simulink model "cvoo_g19_at_sens_est_bombom"  (R2020a)
settings: Solver=VariableStepAuto  StartTime=0.0  StopTime=100  RelTol=1e-3
values from neighbouring files (symbols this model uses):
  b_h_pt = [ ... (first row only)    [main.m]
  c_h_pt = eye(size(a_h_pt))    [main.m]
  conv_max = 5    [main.m]
  conv_min = 0    [main.m]
  conv_rms = 1.5*conv_res    (= 0.000915639116103)    [main.m]
  d_h_pt = zeros(size(b_h_pt))    [main.m]
  deg = pi/180    (= 0.0174532925199)    [main.m]    (also in main_gaspar.m)
  f_amost = 100    [main.m]
  fat_conv_ra = 1/3    (= 0.333333333333)    [main.m]
  G_ra = 10e-3/ft    (= 0.0328083989501)    [main.m]
  G_sensq = (V_max_sensq-V_min_sensq)/(q_max_sensq-q_min_sensq)    (= 0.006)    [main.m]
  Gp_din = (v_pdin_max-v_pdin_min)/(pdin_max-pdin_min)    (= 0.00125)    [main.m]
  h_pt_ref = -1    [main.m]    (also in main_gaspar.m)
  h_ra_max = 1500*ft    (= 457.2)    [main.m]
  h_ra_min = 0    [main.m]
  h_ref = fscanf(fileID,'    [ground_model.m]
  K_lqr = lqr(a_h_pt_int, b_h_pt_int, Q, R)    [main.m]    (also in main_gaspar.m = lqr(a_h_int, b_h_sf_int, Q, R))
  offset_alt = 200    [main.m]
  offset_pdin = 2.5    [main.m]
  Offset_ra = 0    [main.m]
  Offset_sensq = 2.5    [main.m]
  p_din_tau = 0.01    [main.m]
  pdin_max = 2e3    (= 2000)    [main.m]
  pdin_min = -2e3    (= -2000)    [main.m]
  q_max_sensq = 300    [main.m]
  q_min_sensq = -300    [main.m]
  ra_rms = 0.015    [main.m]
  rad = 180/pi    (= 57.2957795131)    [main.m]    (also in main_gaspar.m)
  rho0 = 1.225    [main.m]
  rms_sensq = 4.4    [main.m]
  tau = 0.1    [main.m]
  u_ref = 2    [main.m]    (also in main_gaspar.m = -5)
  vel_max_at = 60    [main.m]
  x0 = [0 0 0 0]    [main.m]    (also in main_gaspar.m)
  x0_e = [0 0 0 0 0]    [main.m]
undefined symbols (not defined in the file or in its folder): a_h_pt, ae, be, ce, cond_ini, de, max_deflec
libraries: simulink x5
settings Model: Creator=josem  LastModifiedBy=thomasmchilds

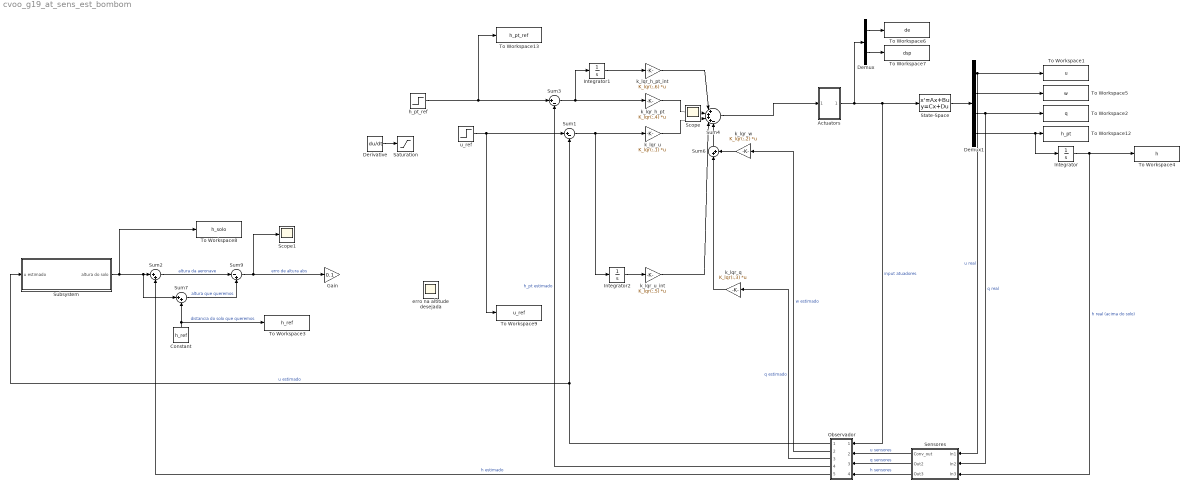
== system cvoo_g19_at_sens_est_bombom ==
  Actuators : Subsystem
  Constant : Constant  Value=h_ref
  Demux : Demux  Outputs=2
  Demux1 : Demux
  Derivative : Derivative
  Gain : Gain  Gain=0.1
  Integrator : Integrator  InitialCondition=cond_ini.h0
  Integrator1 : Integrator
  Integrator2 : Integrator
  Observador : Subsystem
  Saturation : Saturate  UpperLimit=10  LowerLimit=-10
  Scope1 : Scope
  Sensores : Subsystem
  State-Space : StateSpace  A=a_h_pt  B=b_h_pt  C=c_h_pt  D=d_h_pt  InitialCondition=x0
  Subsystem : Subsystem
  Sum1 : Sum  Inputs=|+-
  Sum2 : Sum  Inputs=|++
  Sum3 : Sum  Inputs=|+-
  Sum4 : Sum  Inputs=|++++-
  Sum6 : Sum  Inputs=|++
  Sum7 : Sum  Inputs=|++
  Sum9 : Sum  Inputs=|-+
  To Workspace1 : ToWorkspace  VariableName=u  SampleTime=-1
  To Workspace12 : ToWorkspace  VariableName=h_pt  SampleTime=-1
  To Workspace13 : ToWorkspace  VariableName=h_pt_ref  SampleTime=-1
  To Workspace2 : ToWorkspace  VariableName=q  SampleTime=-1
  To Workspace3 : ToWorkspace  VariableName=h_ref  SampleTime=-1
  To Workspace4 : ToWorkspace  VariableName=h  SampleTime=-1
  To Workspace5 : ToWorkspace  VariableName=w  SampleTime=-1
  To Workspace6 : ToWorkspace  VariableName=de  SaveFormat=Structure With Time  SampleTime=-1
  To Workspace7 : ToWorkspace  VariableName=dsp  SaveFormat=Structure With Time  SampleTime=-1
  To Workspace8 : ToWorkspace  VariableName=h_solo  SampleTime=-1
  To Workspace9 : ToWorkspace  VariableName=u_ref  SampleTime=-1
  erro na altitude desejada : Scope
  h_pt_ref : Step  Time=10  After=h_pt_ref  SampleTime=0  VectorParams1D=off
  k_lqr_h_pt : Gain  Gain=K_lqr(:,4)  Multiplication=Matrix(K*u)
  k_lqr_h_pt_int : Gain  Gain=K_lqr(:,6)  Multiplication=Matrix(K*u)
  k_lqr_q : Gain  Gain=K_lqr(:,3)  Multiplication=Matrix(K*u)
  k_lqr_u : Gain  Gain=K_lqr(:,1)  Multiplication=Matrix(K*u)
  k_lqr_u_int : Gain  Gain=K_lqr(:,5)  Multiplication=Matrix(K*u)
  k_lqr_w : Gain  Gain=K_lqr(:,2)  Multiplication=Matrix(K*u)
  u_ref : Step  Time=50  After=u_ref  SampleTime=0  VectorParams1D=off
  Scope : Scope
  wires:
  State-Space/1 -> Demux1/1
  Demux1/2 -> To Workspace5/1
  k_lqr_h_pt/1 -> Sum4/2
  k_lqr_w/1 -> Sum6/2
  k_lqr_q/1 -> Sum6/1
  Sum6/1 -> Sum4/5
  Demux/1 -> To Workspace6/1
  Demux/2 -> To Workspace7/1
  Demux1/4 -> Integrator/1, To Workspace12/1
  Demux1/1 -> To Workspace1/1, Sensores/1(In1)  "u real"
  k_lqr_u/1 -> Sum4/3
  Sum3/1 -> Integrator1/1, k_lqr_h_pt/1
  Integrator1/1 -> k_lqr_h_pt_int/1
  k_lqr_h_pt_int/1 -> Sum4/1
  k_lqr_u_int/1 -> Sum4/4
  Sum1/1 -> Integrator2/1, k_lqr_u/1
  Integrator2/1 -> k_lqr_u_int/1
  Sum4/1 -> Actuators/1(In1)
  Actuators/1(Out1) -> State-Space/1, Observador/1(In1), Demux/1  "input atuadores"
  Demux1/3 -> To Workspace2/1, Sensores/2(In2)  "q real"
  u_ref/1 -> To Workspace9/1, Sum1/1
  Integrator/1 -> Sensores/3(In3), To Workspace4/1  "h real (acima do solo)"
  Observador/1(Out4) -> Subsystem/1(u estimado), Sum1/2  "u estimado"
  Observador/4(Out1) -> Sum3/2  "h_pt estimado"
  Observador/2(Out2) -> k_lqr_w/1  "w estimado"
  Observador/3(Out3) -> k_lqr_q/1  "q estimado"
  Sensores/1(Conv_out) -> Observador/2(In2)  "u sensores"
  Sensores/2(Out2) -> Observador/3(In3)  "q sensores"
  Sensores/3(Out3) -> Observador/4(In4)  "h sensores"
  Observador/5(Out5) -> Sum2/2  "h estimado"
  Derivative/1 -> Saturation/1
  Sum9/1 -> Scope1/1, Gain/1  "erro de altura abs"
  Sum2/1 -> Sum9/1  "altura da aeronave"
  Subsystem/1(altura do solo) -> To Workspace8/1, Sum7/1, Sum2/1
  Constant/1 -> Sum7/2, To Workspace3/1  "distancia do solo que queremos"
  Sum7/1 -> Sum9/2  "altura que queremos"
  h_pt_ref/1 -> To Workspace13/1, Sum3/1

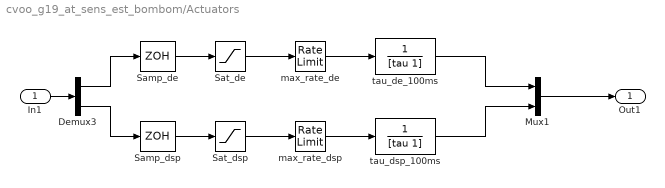
== system cvoo_g19_at_sens_est_bombom/Actuators ==
  In1 : Inport
  " max_rate_de" : RateLimiter  RisingSlewLimit=vel_max_at*deg  FallingSlewLimit=-vel_max_at*deg  SampleTimeMode=inherited
  " max_rate_dsp" : RateLimiter  RisingSlewLimit=vel_max_at*deg  FallingSlewLimit=-vel_max_at*deg  SampleTimeMode=inherited
  Demux3 : Demux  Outputs=2
  Mux1 : Mux  Inputs=2
  Samp_de : ZeroOrderHold  SampleTime=1/f_amost
  Samp_dsp : ZeroOrderHold  SampleTime=1/f_amost
  Sat_de : Saturate  UpperLimit=max_deflec.demax  LowerLimit=max_deflec.demin
  Sat_dsp : Saturate  UpperLimit=max_deflec.spmax  LowerLimit=0
  tau_de_100ms : TransferFcn  Denominator=[tau 1]
  tau_dsp_100ms : TransferFcn  Denominator=[tau 1]
  Out1 : Outport
  wires:
  Mux1/1 -> Out1/1
  In1/1 -> Demux3/1
  Sat_dsp/1 -> " max_rate_dsp"/1
  Sat_de/1 -> " max_rate_de"/1
  Demux3/1 -> Samp_de/1
  Demux3/2 -> Samp_dsp/1
  Samp_dsp/1 -> Sat_dsp/1
  Samp_de/1 -> Sat_de/1
  " max_rate_de"/1 -> tau_de_100ms/1
  " max_rate_dsp"/1 -> tau_dsp_100ms/1
  tau_dsp_100ms/1 -> Mux1/2
  tau_de_100ms/1 -> Mux1/1

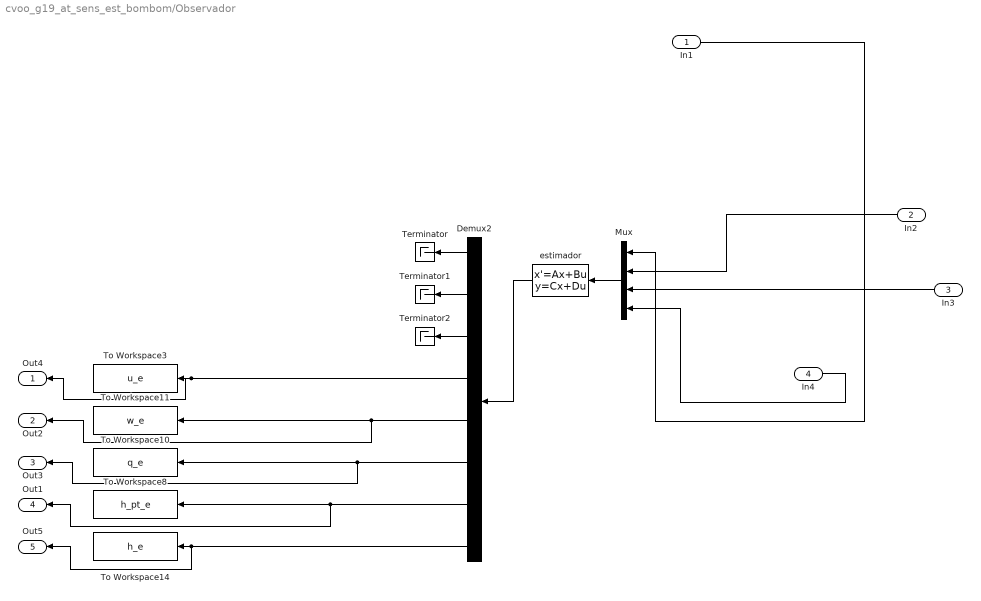
== system cvoo_g19_at_sens_est_bombom/Observador ==
  In1 : Inport
  In2 : Inport  Port=2
  In3 : Inport  Port=3
  In4 : Inport  Port=4
  Demux2 : Demux  Outputs=8
  Mux : Mux
  Terminator : Terminator
  Terminator1 : Terminator
  Terminator2 : Terminator
  To Workspace10 : ToWorkspace  VariableName=q_e  SampleTime=-1
  To Workspace11 : ToWorkspace  VariableName=w_e  SampleTime=-1
  To Workspace14 : ToWorkspace  VariableName=h_e  SampleTime=-1
  To Workspace3 : ToWorkspace  VariableName=u_e  SampleTime=-1
  To Workspace8 : ToWorkspace  VariableName=h_pt_e  SampleTime=-1
  estimador : StateSpace  A=ae  B=be  C=ce  D=de  InitialCondition=x0_e
  Out4 : Outport
  Out2 : Outport  Port=2
  Out3 : Outport  Port=3
  Out1 : Outport  Port=4
  Out5 : Outport  Port=5
  wires:
  Demux2/2 -> Terminator1/1
  estimador/1 -> Demux2/1
  Demux2/5 -> Out2/1, To Workspace11/1
  Demux2/7 -> Out1/1, To Workspace8/1
  Demux2/8 -> Out5/1, To Workspace14/1
  Demux2/1 -> Terminator/1
  Demux2/4 -> Out4/1, To Workspace3/1
  Demux2/3 -> Terminator2/1
  Mux/1 -> estimador/1
  Demux2/6 -> Out3/1, To Workspace10/1
  In1/1 -> Mux/1
  In3/1 -> Mux/3
  In2/1 -> Mux/2
  In4/1 -> Mux/4

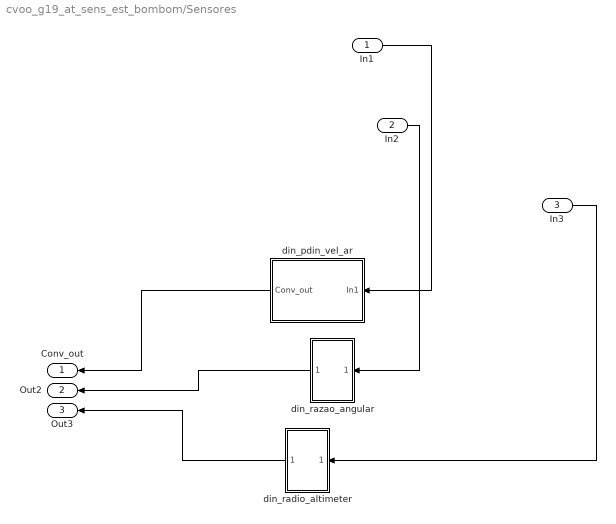
== system cvoo_g19_at_sens_est_bombom/Sensores ==
  In1 : Inport
  In2 : Inport  Port=2
  In3 : Inport  Port=3
  din_pdin_vel_ar : Subsystem
  din_radio_altimeter : Subsystem
  din_razao_angular : Subsystem
  Conv_out : Outport
  Out2 : Outport  Port=2
  Out3 : Outport  Port=3
  wires:
  din_razao_angular/1(Out1) -> Out2/1
  In1/1 -> din_pdin_vel_ar/1(In1)
  din_pdin_vel_ar/1(Conv_out) -> Conv_out/1
  In2/1 -> din_razao_angular/1(In1)
  In3/1 -> din_radio_altimeter/1(In1)
  din_radio_altimeter/1(Out1) -> Out3/1

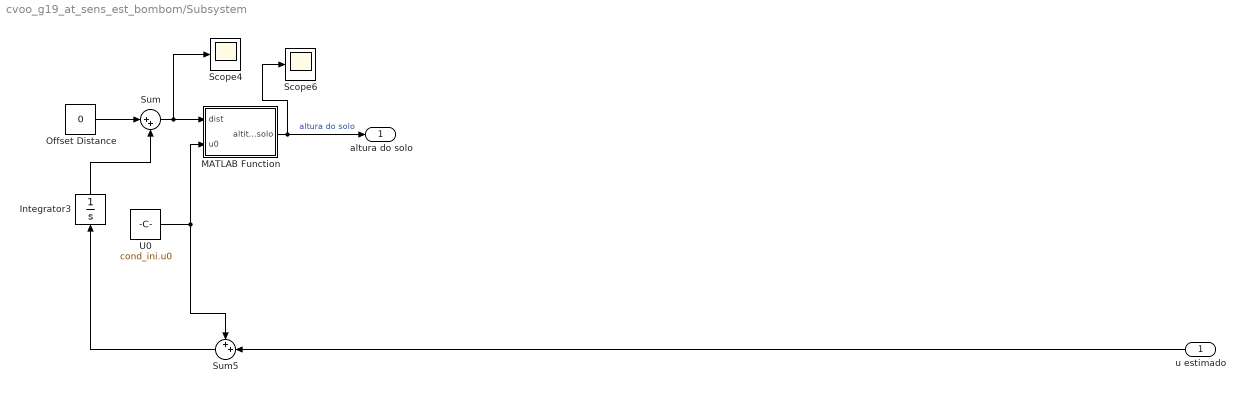
== system cvoo_g19_at_sens_est_bombom/Subsystem ==
  u estimado : Inport
  Integrator3 : Integrator
  MATLAB Function : MATLAB Function  TreatAsAtomicUnit=on
  Offset Distance : Constant  Value=0
  Scope4 : Scope
  Scope6 : Scope
  Sum : Sum  Inputs=|++
  Sum5 : Sum  Inputs=++|
  U0 : Constant  Value=cond_ini.u0
  altura do solo : Outport
  wires:
  Integrator3/1 -> Sum/2
  MATLAB Function/1(altitude_solo) -> altura do solo/1, Scope6/1  "altura do solo"
  Sum5/1 -> Integrator3/1
  U0/1 -> MATLAB Function/2(u0), Sum5/1
  Sum/1 -> Scope4/1, MATLAB Function/1(dist)
  u estimado/1 -> Sum5/2
  Offset Distance/1 -> Sum/1

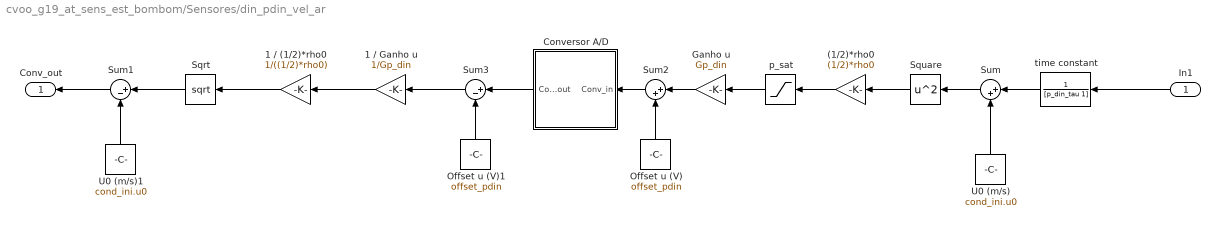
== system cvoo_g19_at_sens_est_bombom/Sensores/din_pdin_vel_ar ==
  In1 : Inport
  " time constant" : TransferFcn  Denominator=[p_din_tau 1]
  (1/2)*rho0 : Gain  Gain=(1/2)*rho0
  1 / (1/2)*rho0 : Gain  Gain=1/((1/2)*rho0)
  1 / Ganho u : Gain  Gain=1/Gp_din
  Conversor A/D : Subsystem
  Ganho u : Gain  Gain=Gp_din
  Offset u (V) : Constant  Value=offset_pdin
  Offset u (V)1 : Constant  Value=offset_pdin
  Sqrt : Sqrt  SaturateOnIntegerOverflow=on
  Square : Math  Operator=square  SignedPower=on  SaturateOnIntegerOverflow=on
  Sum : Sum  Inputs=|++
  Sum1 : Sum  Inputs=|+-
  Sum2 : Sum  Inputs=|++
  Sum3 : Sum  Inputs=|+-
  U0 (m/s) : Constant  Value=cond_ini.u0
  U0 (m/s)1 : Constant  Value=cond_ini.u0
  p_sat : Saturate  UpperLimit=pdin_max  LowerLimit=pdin_min
  Conv_out : Outport
  wires:
  In1/1 -> " time constant"/1
  Sum/1 -> Square/1
  Ganho u/1 -> Sum2/1
  Offset u (V)/1 -> Sum2/2
  " time constant"/1 -> Sum/1
  (1/2)*rho0/1 -> p_sat/1
  U0 (m/s)/1 -> Sum/2
  p_sat/1 -> Ganho u/1
  Square/1 -> (1/2)*rho0/1
  Sum2/1 -> Conversor A/D/1(Conv_in)
  Offset u (V)1/1 -> Sum3/2
  U0 (m/s)1/1 -> Sum1/2
  Sqrt/1 -> Sum1/1
  1 / (1/2)*rho0/1 -> Sqrt/1
  1 / Ganho u/1 -> 1 / (1/2)*rho0/1
  Sum3/1 -> 1 / Ganho u/1
  Conversor A/D/1(Conv_out) -> Sum3/1
  Sum1/1 -> Conv_out/1

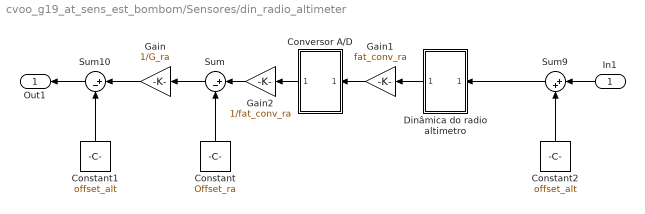
== system cvoo_g19_at_sens_est_bombom/Sensores/din_radio_altimeter ==
  In1 : Inport
  Constant : Constant  Value=Offset_ra
  Constant1 : Constant  Value=offset_alt
  Constant2 : Constant  Value=offset_alt
  Conversor A/D : Subsystem
  Dinâmica do radio altimetro : Subsystem
  Gain : Gain  Gain=1/G_ra
  Gain1 : Gain  Gain=fat_conv_ra
  Gain2 : Gain  Gain=1/fat_conv_ra
  Sum : Sum  Inputs=|+-
  Sum10 : Sum  Inputs=|+-
  Sum9 : Sum  Inputs=|++
  Out1 : Outport
  wires:
  Sum/1 -> Gain/1
  Constant/1 -> Sum/2
  Dinâmica do radio altimetro/1(Out1) -> Gain1/1
  Gain1/1 -> Conversor A/D/1(In1)
  Gain2/1 -> Sum/1
  Conversor A/D/1(Out1) -> Gain2/1
  Constant1/1 -> Sum10/2
  Gain/1 -> Sum10/1
  Sum10/1 -> Out1/1
  Constant2/1 -> Sum9/2
  In1/1 -> Sum9/1
  Sum9/1 -> Dinâmica do radio altimetro/1(In1)

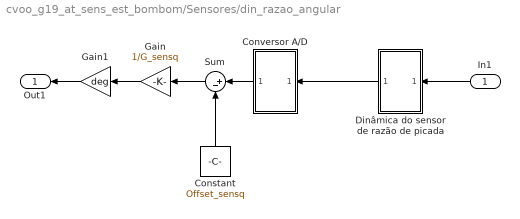
== system cvoo_g19_at_sens_est_bombom/Sensores/din_razao_angular ==
  In1 : Inport
  Constant : Constant  Value=Offset_sensq
  Conversor A/D : Subsystem
  Dinâmica do sensor de razão de picada : Subsystem
  Gain : Gain  Gain=1/G_sensq
  Gain1 : Gain  Gain=deg
  Sum : Sum  Inputs=|+-
  Out1 : Outport
  wires:
  In1/1 -> Dinâmica do sensor de razão de picada/1(In1)
  Dinâmica do sensor de razão de picada/1(Out1) -> Conversor A/D/1(In1)
  Conversor A/D/1(Out1) -> Sum/1
  Sum/1 -> Gain/1
  Constant/1 -> Sum/2
  Gain/1 -> Gain1/1
  Gain1/1 -> Out1/1

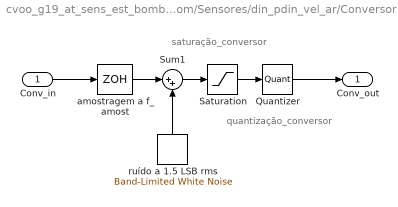
== system cvoo_g19_at_sens_est_bombom/Sensores/din_pdin_vel_ar/Conversor A//D ==
  note: saturação_conversor
  note: quantização_conversor
  Conv_in : Inport
  Quantizer : Quantizer  QuantizationInterval=fat_quant
  Saturation : Saturate  UpperLimit=conv_max  LowerLimit=conv_min
  Sum1 : Sum  Inputs=|++
  amostragem a f_amost : ZeroOrderHold  SampleTime=1/f_amost
  ruído a 1.5 LSB rms : simulink/Sources/Band-Limited White Noise  Cov=[conv_rms^2/f_amost]  Ts=1/f_amost  seed=[23341]
  Conv_out : Outport
  wires:
  Conv_in/1 -> amostragem a f_amost/1
  amostragem a f_amost/1 -> Sum1/1
  ruído a 1.5 LSB rms/1 -> Sum1/2
  Saturation/1 -> Quantizer/1
  Sum1/1 -> Saturation/1
  Quantizer/1 -> Conv_out/1

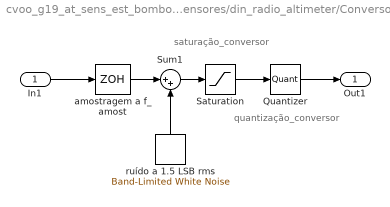
== system cvoo_g19_at_sens_est_bombom/Sensores/din_radio_altimeter/Conversor A//D ==
  note: saturação_conversor
  note: quantização_conversor
  In1 : Inport
  Quantizer : Quantizer  QuantizationInterval=fat_quant
  Saturation : Saturate  UpperLimit=conv_max  LowerLimit=conv_min
  Sum1 : Sum  Inputs=|++
  amostragem a f_amost : ZeroOrderHold  SampleTime=1/f_amost
  ruído a 1.5 LSB rms : simulink/Sources/Band-Limited White Noise  Cov=[conv_rms^2/f_amost]  Ts=1/f_amost  seed=[23341]
  Out1 : Outport
  wires:
  In1/1 -> amostragem a f_amost/1
  amostragem a f_amost/1 -> Sum1/1
  ruído a 1.5 LSB rms/1 -> Sum1/2
  Saturation/1 -> Quantizer/1
  Sum1/1 -> Saturation/1
  Quantizer/1 -> Out1/1

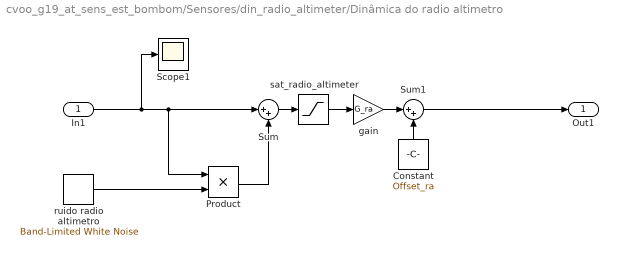
== system cvoo_g19_at_sens_est_bombom/Sensores/din_radio_altimeter/Dinâmica do radio altimetro ==
  In1 : Inport
  Constant : Constant  Value=Offset_ra
  Product : Product
  Scope1 : Scope
  Sum : Sum  Inputs=|++
  Sum1 : Sum  Inputs=|++
  gain : Gain  Gain=G_ra
  ruido radio altimetro : simulink/Sources/Band-Limited White Noise  Cov=[ra_rms^2/f_amost]  Ts=1/f_amost  seed=[23341]
  sat_radio_altimeter : Saturate  UpperLimit=h_ra_max  LowerLimit=h_ra_min
  Out1 : Outport
  wires:
  Sum1/1 -> Out1/1
  Sum/1 -> sat_radio_altimeter/1
  Constant/1 -> Sum1/2
  gain/1 -> Sum1/1
  sat_radio_altimeter/1 -> gain/1
  In1/1 -> Scope1/1, Sum/1, Product/1
  ruido radio altimetro/1 -> Product/2
  Product/1 -> Sum/2

== system cvoo_g19_at_sens_est_bombom/Sensores/din_razao_angular/Conversor A//D ==
  note: saturação_conversor
  note: quantização_conversor
  In1 : Inport
  Quantizer : Quantizer  QuantizationInterval=fat_quant
  Saturation : Saturate  UpperLimit=conv_max  LowerLimit=conv_min
  Sum1 : Sum  Inputs=|++
  amostragem a f_amost : ZeroOrderHold  SampleTime=1/f_amost
  ruído a 1.5 LSB rms : simulink/Sources/Band-Limited White Noise  Cov=[conv_rms^2/f_amost]  Ts=1/f_amost  seed=[23341]
  Out1 : Outport
  wires:
  In1/1 -> amostragem a f_amost/1
  amostragem a f_amost/1 -> Sum1/1
  ruído a 1.5 LSB rms/1 -> Sum1/2
  Saturation/1 -> Quantizer/1
  Sum1/1 -> Saturation/1
  Quantizer/1 -> Out1/1

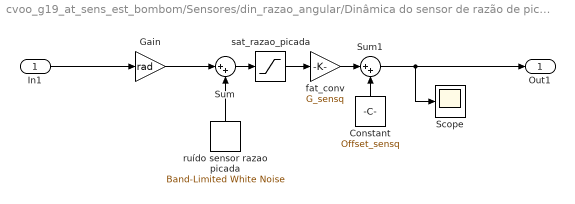
== system cvoo_g19_at_sens_est_bombom/Sensores/din_razao_angular/Dinâmica do sensor de razão de picada ==
  In1 : Inport
  Constant : Constant  Value=Offset_sensq
  Gain : Gain  Gain=rad
  Scope : Scope
  Sum : Sum  Inputs=|++
  Sum1 : Sum  Inputs=|++
  fat_conv : Gain  Gain=G_sensq
  ruído sensor razao picada : simulink/Sources/Band-Limited White Noise  Cov=[rms_sensq^2/f_amost]  Ts=1/f_amost  seed=[23341]
  sat_razao_picada : Saturate  UpperLimit=q_max_sensq  LowerLimit=q_min_sensq
  Out1 : Outport
  wires:
  ruído sensor razao picada/1 -> Sum/2
  Sum1/1 -> Scope/1, Out1/1
  In1/1 -> Gain/1
  Sum/1 -> sat_razao_picada/1
  Constant/1 -> Sum1/2
  fat_conv/1 -> Sum1/1
  sat_razao_picada/1 -> fat_conv/1
  Gain/1 -> Sum/1

== matlab function cvoo_g19_at_sens_est_bombom/Subsystem/MATLAB Function ==
  data: dist input; altitude_solo output; u0 input
function altitude_solo = fcn(dist,u0)

altitude_solo = 5*u0;

if dist >= 0 && dist < 20*u0
    altitude_solo = -dist/4 + 5*u0;
elseif dist >= 20*u0 && dist < 40*u0
    altitude_solo = 0;
elseif dist >= 40*u0 && dist < 60*u0
    %altitude_solo = p(1)*dist^3 + p(2)*dist^2 + p(3)*dist + p(4);
    altitude_solo = 3*u0;
elseif dist >= 60*u0 && dist <= 80*u0
    altitude_solo = 5*u0;
end
